simulink model "e8_2_sim"  (R2016b)
settings: Solver=ode4  StartTime=0.0  StopTime=50  FixedStep=0.001  RelTol=1e-3
InitFcn:
  | Init_control;
values from neighbouring files (symbols this model uses):
  DEG2RAD = 0.0174533    [Init_control.m]
  Kd_PITCH_AgngleRate = 0.001    [Init_control.m]
  Kd_ROLL_AgngleRate = 0.001    [Init_control.m]
  Kd_YAW_AngleRate = 0.00    (= 0)    [Init_control.m]
  Ki_PITCH_AgngleRate = 0.02    [Init_control.m]
  Ki_ROLL_AgngleRate = 0.02    [Init_control.m]
  Ki_YAW_AngleRate = 0.01    [Init_control.m]
  Kp_PITCH_AgngleRate = 0.1    [Init_control.m]
  Kp_PITCH_ANGLE = 6.5    [Init_control.m]
  Kp_ROLL_AgngleRate = 0.1    [Init_control.m]
  Kp_ROLL_ANGLE = 6.5    [Init_control.m]
  Kp_YAW_AngleRate = 0.5    [Init_control.m]
  Kpxp = 1.0    (= 1)    [Init_control.m]
  Kpyp = 1.0    (= 1)    [Init_control.m]
  Kpzp = 4.0    (= 4)    [Init_control.m]
  Kvxd = 0.01    [Init_control.m]
  Kvxi = 0.1    [Init_control.m]
  Kvxp = 3.0    (= 3)    [Init_control.m]
  Kvyd = 0.01    [Init_control.m]
  Kvyi = 0.1    [Init_control.m]
  Kvyp = 3.0    (= 3)    [Init_control.m]
  Kvzd = 0.005    [Init_control.m]
  Kvzi = 0.01    [Init_control.m]
  Kvzp = 0.45    [Init_control.m]
  MAX_CONTROL_ANGLE_PITCH = 35    [Init_control.m]
  MAX_CONTROL_ANGLE_RATE_PITCH = 220    [Init_control.m]
  MAX_CONTROL_ANGLE_RATE_ROLL = 220    [Init_control.m]
  MAX_CONTROL_ANGLE_RATE_Y = 200    [Init_control.m]
  MAX_CONTROL_ANGLE_ROLL = 35    [Init_control.m]
  MAX_CONTROL_VELOCITY_XY = 5    [Init_control.m]
  MAX_CONTROL_VELOCITY_Z = 3    [Init_control.m]
  ModelInit_AngEuler = [0,0,0]    [Init_control.m]
  ModelInit_PosE = [0,0,0]    [Init_control.m]
  ModelInit_RateB = [0,0,0]    [Init_control.m]
  ModelInit_RPM = 0    [Init_control.m]
  ModelInit_VelB = [0,0,0]    [Init_control.m]
  Saturation_I_ah = 3.43    [Init_control.m]
  Saturation_I_az = 5    [Init_control.m]
  Saturation_I_RP_Max = 0.3    [Init_control.m]
  Saturation_I_RP_Min = -0.3    [Init_control.m]
  Saturation_I_Y_Max = 0.2    [Init_control.m]
  Saturation_I_Y_Min = -0.2    [Init_control.m]
  THR_HOVER = 0.609    [Init_control.m]
undefined symbols (not defined in the file or in its folder): DiscIntNeverNeededParam, earthRadius, KiRollAttitude, ModelParam_envGravityAcc, ModelParam_motorCr, ModelParam_motorJm, ModelParam_motorT, ModelParam_motorWb, ModelParam_rotorCm, ModelParam_rotorCt, ModelParam_uavCd, ModelParam_uavJ, ModelParam_uavMass, ModelParam_uavR
libraries: simulink x10, aerolibutil x2, aerolibfltsims x2, aerolibanimutils x1
(part 2 of 2)

== matlab function e8_2_sim/Control System/MATLAB Function1 ==
  data: state input; vxd output; vyd output; vzd output; x input; y input; z input; vx input; vy input; vz input; xd output; yd output; zd output
function [vxd,vyd,vzd,xd,yd,zd] = fcn(state,x,y,z,vx,vy,vz)
persistent hold_x_flag;
if isempty(hold_x_flag)
    hold_x_flag=0;
end
persistent hold_y_flag;
if isempty(hold_y_flag)
    hold_y_flag=0;
end
persistent hold_z_flag;
if isempty(hold_z_flag)
    hold_z_flag=0;
end
persistent x1;
if isempty(x1)
    x1=0;
end
persistent y1;
if isempty(y1)
    y1=0;
end

persistent z1;
if isempty(z1)
    z1=0;
end

heightSafe=50;
if state==1 %返航，高度低于指定阈值，先上升到指定值
    vxd=0;%将水平速度降为0
    vyd=0;
    if abs(z)<heightSafe
        z1=-heightSafe;vzd=0;%期望高度设为50
        hold_z_flag = 0;
    else
        vzd = 0;
        if abs(vz)< 6 &&(hold_z_flag<0.5)
            z1 = z; 
            hold_z_flag=1;
        end
        if ~(abs(vz)<6)
           z1=z;
           hold_z_flag = 0;
        end
    end
    
    if abs(vx) < 8 && (hold_x_flag < 0.5)
       x1 = 0; 
       hold_x_flag = 1;
   end
   if ~(abs(vx) < 8)
       x1 = x; 
       hold_x_flag = 0;
   end
   if abs(vy)< 8 && (hold_y_flag < 0.5)
       y1 = 0;
       hold_y_flag = 1;
   end
   if ~(abs(vy) < 8)
       y1 = y;
       hold_y_flag = 0;
   end
elseif state==2%着陆
    vxd = 0; vyd = 0;
   z1 = 0;vzd = 0;%期望高度为0，进行着陆
   hold_z_flag = 0;
   %解决漂移问题
   if abs(vx) < 8 && (hold_x_flag < 0.5)
       x1 = x; 
       hold_x_flag = 1;
   end
   if ~(abs(vx) < 8)
       x1 = x; 
       hold_x_flag = 0;
   end
   if abs(vy) < 8 && (hold_y_flag < 0.5)
       y1 = y;
       hold_y_flag = 1;
   end
   if ~(abs(vy)<8)
       y1=y;
       hold_y_flag=0;
   end
   
else%手动
   x1 = x; vxd = 0;
   y1 = y; vyd = 0;
   z1 = z; vzd = 0;
   
   hold_x_flag = 0;
   hold_y_flag = 0;
   hold_z_flag = 0;
end

 xd=x1;
 yd=y1;
 zd=z1;
